simulink model "VSG_2M"  (R2022b)
settings: Solver=FixedStepAuto  StartTime=0.0  StopTime=2  FixedStep=1e-6  RelTol=1e-3
model workspace (MAT data in the model file):
  C = 0.0003
  D = 500
  GP = 0.6
  GQ = 20
  J = 2
  KQ = 0.06
  Kf = 80000
  Kv = 577
  L = 0.001
  Pref = 2000000
  Qref = 0
  Ts = 0.0001
  Ts_Power = 1e-06
  Ug = 400
  Vdc = 1000
  fsw = 20000
  t0 = 0.5
  tco = 1.3
  tf = 1.2
  wn = 314.159265359
undefined symbols (not defined in the file): DiscIntNeverNeededParam, Ion, Lithium
libraries: spsSeriesRLCBranchLib x8, spsFirstOrderFilterLib x7, spsMeanLib x5, slpidlib x5, spsabctodq0Lib x4, spsStairGeneratorLib x4, spsDiodeLib x4, spsPWMGeneratorDCDCLib x3, spsThreePhaseVIMeasurementLib x3, spsThreePhaseSeriesRLCBranchLib x3, spsPowerPositiveSequenceLib x2, spsBoostConverterLib x2
(part 1 of 2)
settings Model: SimulationMode=accelerator  Creator=刘明炜  LastModifiedBy=刘明炜
settings DataIOCC: ReturnWorkspaceOutputs=off

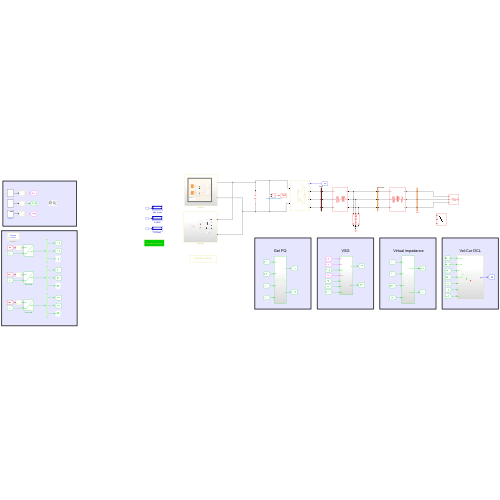
[thumbnail: Simulink's stored preview of the top-level diagram]
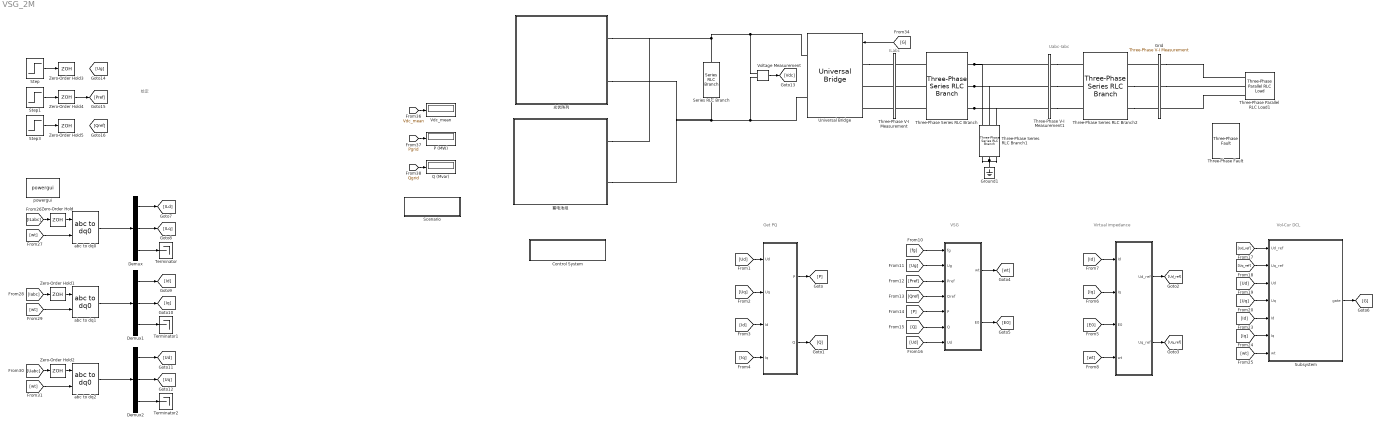
== system VSG_2M ==
  note: 给定
  note: ILabc
  note: VSG
  note: Get PQ
  note: Virtual impedance
  note: Vol-Cur DCL
  note: Uabc-Iabc
  " " : Subsystem
  "  " : Subsystem
  "   " : Subsystem
  Control System : Subsystem
      mask Display: disp('CONTROL SYSTEM')
  Demux : Demux  Outputs=3
  Demux1 : Demux  Outputs=3
  Demux2 : Demux  Outputs=3
  Grid : spsThreePhaseVIMeasurementLib/Three-Phase V-I Measurement  VoltageMeasurement=phase-to-ground  SetLabelV=on  LabelV=Vgrid  Vpu=off  VpuLL=off  CurrentMeasurement=yes  SetLabelI=on  LabelI=Igrid  Ipu=off  Pbase=100e6  Vbase=500e3  OutputType=Complex  PhasorSimulation=off  PSBequivalent=0
  Ground1 : spsGroundLib/Ground  LConnTagsString=a
  P (MW) : Display
      settings: Format=bank  Decimation=200
  Q (Mvar) : Display
      settings: Format=bank  Decimation=200
  Scenario : Subsystem
      mask Display: disp('Scenario & Scopes')
  Series RLC Branch : spsSeriesRLCBranchLib/Series RLC Branch  LConnTagsString=__new0  RConnTagsString=__new0  BranchType=C  Resistance=1  Inductance=1e-3  SetiL0=off  InitialCurrent=0  Capacitance=0.47  Setx0=off  InitialVoltage=0  Measurements=None
  Step : Step  Time=t0  Before=1  After=Ug  SampleTime=0
  Step1 : Step  Time=0  After=Pref  SampleTime=0
  Step3 : Step  Time=0  After=Qref  SampleTime=0
  Subsystem : Subsystem
  Terminator : Terminator
  Terminator1 : Terminator
  Terminator2 : Terminator
  Three-Phase Parallel RLC Load1 : spsThreePhaseParallelRLCLoadLib/Three-Phase Parallel RLC Load  LConnTagsString=A|B|C  Configuration=Y (grounded)  NominalVoltage=400  Vabc=[1e3 1e3 1e3]  Vabcp=[1e3 1e3 1e3]  NominalFrequency=50  UnbalancedPower=off  ActivePower=Pref  InductivePower=0  CapacitivePower=0  Pabc=[10e3 9e3 11e3]  QLabc=[100 90 110]  QCabc=[100 90 110]  Pabcp=[10e3 9e3 11e3]  QLabcp=[100 90 110]  QCabcp=[100 90 110]  Measurements=Branch voltages and currents  LoadType=constant Z
  Three-Phase Series RLC Branch : spsThreePhaseSeriesRLCBranchLib/Three-Phase Series RLC Branch  LConnTagsString=A|B|C  RConnTagsString=A|B|C  BranchType=RL  Resistance=0  Inductance=L  Capacitance=0  Measurements=None
  Three-Phase Series RLC Branch1 : spsThreePhaseSeriesRLCBranchLib/Three-Phase Series RLC Branch  LConnTagsString=A|B|C  RConnTagsString=A|B|C  BranchType=RLC  Resistance=1  Inductance=0  Capacitance=C  Measurements=None
  Three-Phase Series RLC Branch2 : spsThreePhaseSeriesRLCBranchLib/Three-Phase Series RLC Branch  LConnTagsString=A|B|C  RConnTagsString=A|B|C  BranchType=RLC  Resistance=0  Inductance=0.00000001  Capacitance=0  Measurements=None
  Three-Phase V-I Measurement : spsThreePhaseVIMeasurementLib/Three-Phase V-I Measurement  VoltageMeasurement=phase-to-phase  SetLabelV=on  LabelV=Vinv  Vpu=off  VpuLL=off  CurrentMeasurement=yes  SetLabelI=on  LabelI=ILabc  Ipu=off  Pbase=100e6  Vbase=500e3  OutputType=Complex  PhasorSimulation=off  PSBequivalent=0
  Three-Phase V-I Measurement1 : spsThreePhaseVIMeasurementLib/Three-Phase V-I Measurement  VoltageMeasurement=phase-to-ground  SetLabelV=on  LabelV=Uabc  Vpu=off  VpuLL=off  CurrentMeasurement=yes  SetLabelI=on  LabelI=Iabc  Ipu=off  Pbase=100e6  Vbase=500e3  OutputType=Complex  PhasorSimulation=off  PSBequivalent=0
  Three-Phase Fault : spsThreePhaseFaultLib/Three-Phase Fault  InitialStates=0  FaultA=on  FaultB=off  FaultC=off  GroundFault=on  SwitchTimes=[tf tco]  External=off  SwitchStatus=NaN  FaultResistance=1  GroundResistance=0.01  SnubberResistance=1e6  SnubberCapacitance=inf  Measurements=Fault voltages and currents
  Universal Bridge : spsUniversalBridgeLib/Universal Bridge  Arms=3  SnubberResistance=1e5  SnubberCapacitance=inf  Device=IGBT / Diodes  Ron=0.001  Lon=0  ForwardVoltages="[  0  0  ]"  ForwardVoltage=0  GTOparameters=[ 10e-6 , 20e-6 ]  IGBTparameters=[ 1e-6 , 2e-6 ]  Measurements=None  Measurements_2=None  converterType=Rectifier
  Vdc_mean : Display
      settings: Decimation=200
  Voltage Measurement : spsVoltageMeasurementLib/Voltage Measurement  PhasorSimulation=off  OutputType=Complex  PSBequivalent=0
  Zero-Order Hold{,1..5} (6 alike) : ZeroOrderHold  SampleTime=1/fsw
  abc to dq0 : spsabctodq0Lib/abc to dq0  Alignment=90 degrees behind phase A axis
  abc to dq1 : spsabctodq0Lib/abc to dq0  Alignment=90 degrees behind phase A axis
  abc to dq2 : spsabctodq0Lib/abc to dq0  Alignment=90 degrees behind phase A axis
  powergui : spspowerguiLib/powergui  Priority=1  SimulationMode=Discrete  SampleTime=Ts_Power  frequency=60  Iterations=50  frequencyindice=0  Pbase=100e6  ErrMax=1e-4  UnitsV=kV  UnitsW=MW  buscounter=0  FunctionMessages=off  echomessages=off  EnableUseOfTLC=off  CurrentSourceSwitches=off  DisableSnubberDevices=off  DisableRonSwitches=off  DisableVfSwitches=off  DisplayEquations=off  AutomaticDiscreteSolvers=off  SolverType=Tustin/Backward Euler (TBE)  Interpol=off  ExternalGateDelay=off  methode=off  Ts=100  x0status=blocks  SPID=on  SwTol=0  HookPort=off  NonlinearTolerance=1e-4  nMaxIteration=100  ContinueOnMaxIteration=off  RestoreLinks=warning  ResistiveCurrentMeasurement=off  Frange=[0:2:500]  Ylog=off  Xlog=on  ShowGrid=off  save=off  variable=ZData  structure=0  ZoomFFT=off  StartTime=0.0  cycles=1  DisplayStyle=1  fundamental=60  FreqAxis=off  MaxFrequency=1000  frequencyindicesteady=1  RmsSteady=1  display=off
  光伏阵列 : Subsystem
  蓄电池组 : Subsystem
  wires:
  [Id] -> " "/3(Id)
  [Iq] -> " "/4(Iq)
  [Uq] -> " "/2(Uq)
  " "/1(P) -> [P]
  [Ud] -> " "/1(Ud)
  " "/2(Q) -> [Q]
  [E0] -> "   "/3(E0)
  [Iq] -> "   "/2(Iq)
  [Id] -> "   "/1(Id)
  [wt] -> "   "/4(wt)
  "   "/1(Ud_ref) -> [Ud_ref]
  "   "/2(Uq_ref) -> [Uq_ref]
  [Qref] -> "  "/4(Qref)
  [Ud] -> "  "/7(Ud)
  [fg] -> "  "/1(fg)
  "  "/2(E0) -> [E0]
  [Q] -> "  "/6(Q)
  [P] -> "  "/5(P)
  [Ug] -> "  "/2(Ug)
  [Pref] -> "  "/3(Pref)
  "  "/1(wt) -> [wt]
  [Ud] -> Subsystem/3(Ud)
  Subsystem/1(gate) -> [G]
  [wt] -> Subsystem/7(wt)
  [Ud_ref] -> Subsystem/1(Ud_ref)
  [Uq_ref] -> Subsystem/2(Uq_ref)
  [Iq] -> Subsystem/6(Iq)
  [Uq] -> Subsystem/4(Uq)
  [Id] -> Subsystem/5(Id)
  abc to dq0/1 -> Demux/1
  Demux/1 -> [ILd]
  Demux/2 -> [ILq]
  Demux/3 -> Terminator/1
  Demux1/2 -> [Iq]
  Demux1/1 -> [Id]
  abc to dq1/1 -> Demux1/1
  Demux1/3 -> Terminator1/1
  Demux2/2 -> [Uq]
  Demux2/1 -> [Ud]
  abc to dq2/1 -> Demux2/1
  Demux2/3 -> Terminator2/1
  Zero-Order Hold/1 -> abc to dq0/1
  [ILabc] -> Zero-Order Hold/1
  [Iabc] -> Zero-Order Hold1/1
  Zero-Order Hold1/1 -> abc to dq1/1
  [Uabc] -> Zero-Order Hold2/1
  Zero-Order Hold2/1 -> abc to dq2/1
  [wt] -> abc to dq0/2
  [wt] -> abc to dq1/2
  [wt] -> abc to dq2/2
  Step/1 -> Zero-Order Hold3/1
  Step1/1 -> Zero-Order Hold4/1
  [G] -> Universal Bridge/1
  Step3/1 -> Zero-Order Hold5/1
  [Qgrid] -> Q (Mvar)/1
  [Pgrid] -> P (MW)/1
  [Vdc_mean] -> Vdc_mean/1
  Voltage Measurement/1 -> [Vdc]
  Zero-Order Hold4/1 -> [Pref]
  connections:
  Three-Phase Series RLC Branch/RConn1 -- Three-Phase Series RLC Branch1/LConn1 -- Three-Phase V-I Measurement1/LConn1
  Ground1/LConn1 -- Three-Phase Series RLC Branch1/RConn2 -- Three-Phase Series RLC Branch1/RConn3 -- Three-Phase Series RLC Branch1/RConn1
  Three-Phase Series RLC Branch/RConn3 -- Three-Phase V-I Measurement1/LConn3 -- Three-Phase Series RLC Branch1/LConn3
  Three-Phase Series RLC Branch/RConn2 -- Three-Phase Series RLC Branch1/LConn2 -- Three-Phase V-I Measurement1/LConn2
  Three-Phase Series RLC Branch/LConn1 -- Three-Phase V-I Measurement/RConn1
  Three-Phase V-I Measurement1/RConn3 -- Three-Phase Series RLC Branch2/LConn3
  Three-Phase V-I Measurement/LConn2 -- Universal Bridge/LConn2
  Universal Bridge/RConn2 -- Voltage Measurement/LConn2 -- 蓄电池组/RConn2 -- 光伏阵列/RConn2 -- Series RLC Branch/RConn1
  Universal Bridge/LConn1 -- Three-Phase V-I Measurement/LConn1
  Three-Phase V-I Measurement1/RConn2 -- Three-Phase Series RLC Branch2/LConn2
  Universal Bridge/RConn1 -- 蓄电池组/RConn1 -- 光伏阵列/RConn1 -- Series RLC Branch/LConn1 -- Voltage Measurement/LConn1
  Three-Phase V-I Measurement1/RConn1 -- Three-Phase Series RLC Branch2/LConn1
  Three-Phase Series RLC Branch/LConn2 -- Three-Phase V-I Measurement/RConn2
  Three-Phase Series RLC Branch/LConn3 -- Three-Phase V-I Measurement/RConn3
  Three-Phase V-I Measurement/LConn3 -- Universal Bridge/LConn3
  Grid/LConn1 -- Three-Phase Series RLC Branch2/RConn1
  Three-Phase Series RLC Branch2/RConn2 -- Grid/LConn2
  Three-Phase Series RLC Branch2/RConn3 -- Grid/LConn3
  Grid/RConn1 -- Three-Phase Parallel RLC Load1/LConn1
  Grid/RConn2 -- Three-Phase Parallel RLC Load1/LConn2
  Three-Phase Parallel RLC Load1/LConn3 -- Grid/RConn3

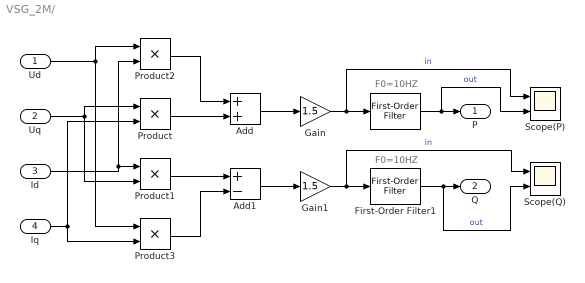
== system VSG_2M/  ==
  note: F0=10HZ
  note: F0=10HZ
  Ud : Inport
  Uq : Inport  Port=2
  Id : Inport  Port=3
  Iq : Inport  Port=4
  " " : spsFirstOrderFilterLib/First-Order Filter  FilterType=Lowpass  Tc=10e-3  Ts=1/fsw  Initialize=on  Vac_Init=[0, 0, 10]  Vdc_Init=0  PlotResponse=off  FreqRange="[0,  200,  1]"
  Add : Sum
  Add1 : Sum  Inputs=+-
  First-Order Filter1 : spsFirstOrderFilterLib/First-Order Filter  FilterType=Lowpass  Tc=10e-3  Ts=1/fsw  Initialize=on  Vac_Init=[0, 0, 10]  Vdc_Init=0  PlotResponse=off  FreqRange="[0,  200,  1]"
  Gain : Gain  Gain=1.5
  Gain1 : Gain  Gain=1.5
  Product{,1..3} (4 alike) : Product
  Scope(P) : Scope  NumInputPorts=2
  Scope(Q) : Scope  NumInputPorts=2
  P : Outport
  Q : Outport  Port=2
  wires:
  Gain1/1 -> First-Order Filter1/1, Scope(Q)/1  "in"
  Product2/1 -> Add/1
  " "/1 -> Scope(P)/2, P/1  "out"
  Add1/1 -> Gain1/1
  Gain/1 -> " "/1, Scope(P)/1  "in"
  First-Order Filter1/1 -> Scope(Q)/2, Q/1  "out"
  Product/1 -> Add/2
  Product3/1 -> Add1/2
  Product1/1 -> Add1/1
  Ud/1 -> Product3/1, Product2/1
  Add/1 -> Gain/1
  Id/1 -> Product1/1, Product2/2
  Iq/1 -> Product3/2, Product/2
  Uq/1 -> Product1/2, Product/1

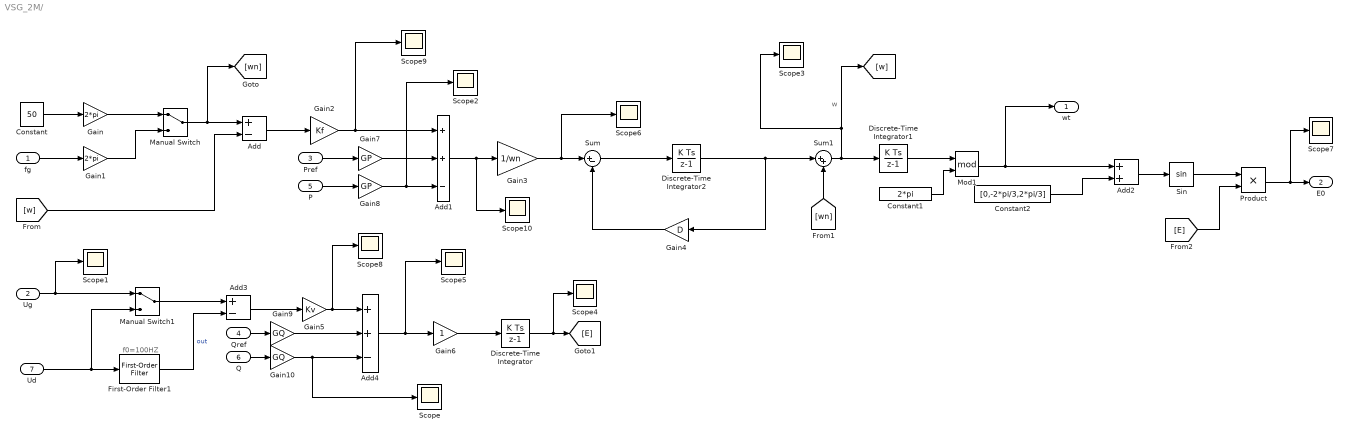
== system VSG_2M/   ==
  note: f0=100HZ
  note: w
  fg : Inport
  Ug : Inport  Port=2
  Pref : Inport  Port=3
  Qref : Inport  Port=4
  P : Inport  Port=5
  Q : Inport  Port=6
  Ud : Inport  Port=7
  Add : Sum  Inputs=+-
  Add1 : Sum  Inputs=++-
  Add2 : Sum
  Add3 : Sum  Inputs=+-
  Add4 : Sum  Inputs=++-
  Constant : Constant  Value=50
  Constant1 : Constant  Value=2*pi
  Constant2 : Constant  Value=[0,-2*pi/3,2*pi/3]
  Discrete-Time Integrator : DiscreteIntegrator  gainval=KQ  SampleTime=1/fsw  ICPrevOutput=DiscIntNeverNeededParam  ICPrevScaledInput=DiscIntNeverNeededParam
  Discrete-Time Integrator1 : DiscreteIntegrator  SampleTime=1/fsw  ICPrevOutput=DiscIntNeverNeededParam  ICPrevScaledInput=DiscIntNeverNeededParam
  Discrete-Time Integrator2 : DiscreteIntegrator  gainval=1/J  SampleTime=1/fsw  ICPrevOutput=DiscIntNeverNeededParam  ICPrevScaledInput=DiscIntNeverNeededParam
  First-Order Filter1 : spsFirstOrderFilterLib/First-Order Filter  FilterType=Lowpass  Tc=10e-3  Ts=1/fsw  Initialize=on  Vac_Init=[0, 0, 10]  Vdc_Init=0  PlotResponse=off  FreqRange="[0,  200,  1]"
  Gain : Gain  Gain=2*pi
  Gain1 : Gain  Gain=2*pi
  Gain10 : Gain  Gain=GQ
  Gain2 : Gain  Gain=Kf
  Gain3 : Gain  Gain=1/wn
  Gain4 : Gain  Gain=D
  Gain5 : Gain  Gain=Kv
  Gain6 : Gain
  Gain7 : Gain  Gain=GP
  Gain8 : Gain  Gain=GP
  Gain9 : Gain  Gain=GQ
  Manual Switch : ManualSwitch
  Manual Switch1 : ManualSwitch
  Mod1 : Math  Operator=mod
  Product : Product
  Scope{,1..10} (11 alike) : Scope
  Sin : Trigonometry
  Sum : Sum  Inputs=|+-
  Sum1 : Sum  Inputs=|++
  wt : Outport
  E0 : Outport  Port=2
  wires:
  Ug/1 -> Scope1/1, Manual Switch1/1
  Gain3/1 -> Scope6/1, Sum/1
  Gain2/1 -> Scope9/1, Add1/1
  Product/1 -> Scope7/1, E0/1
  Add/1 -> Gain2/1
  Manual Switch1/1 -> Add3/1
  [E] -> Product/2
  Add4/1 -> Scope5/1, Gain6/1
  Mod1/1 -> wt/1, Add2/1
  Sum1/1 -> Discrete-Time Integrator1/1, Scope3/1, [w]
  fg/1 -> Gain1/1
  Constant2/1 -> Add2/2
  First-Order Filter1/1 -> Add3/2  "out"
  Ud/1 -> First-Order Filter1/1, Manual Switch1/2
  Constant/1 -> Gain/1
  Sin/1 -> Product/1
  Add2/1 -> Sin/1
  Gain4/1 -> Sum/2
  P/1 -> Gain8/1
  Gain/1 -> Manual Switch/1
  Gain1/1 -> Manual Switch/2
  Discrete-Time Integrator2/1 -> Gain4/1, Sum1/1
  Constant1/1 -> Mod1/2
  Gain5/1 -> Scope8/1, Add4/1
  Q/1 -> Gain10/1
  Manual Switch/1 -> [wn], Add/1
  Pref/1 -> Gain7/1
  Add1/1 -> Scope10/1, Gain3/1
  Add3/1 -> Gain5/1
  Gain6/1 -> Discrete-Time Integrator/1
  Qref/1 -> Gain9/1
  [wn] -> Sum1/2
  Sum/1 -> Discrete-Time Integrator2/1
  Discrete-Time Integrator/1 -> Scope4/1, [E]
  Discrete-Time Integrator1/1 -> Mod1/1
  [w] -> Add/2
  Gain7/1 -> Add1/2
  Gain8/1 -> Scope2/1, Add1/3
  Gain9/1 -> Add4/2
  Gain10/1 -> Scope/1, Add4/3

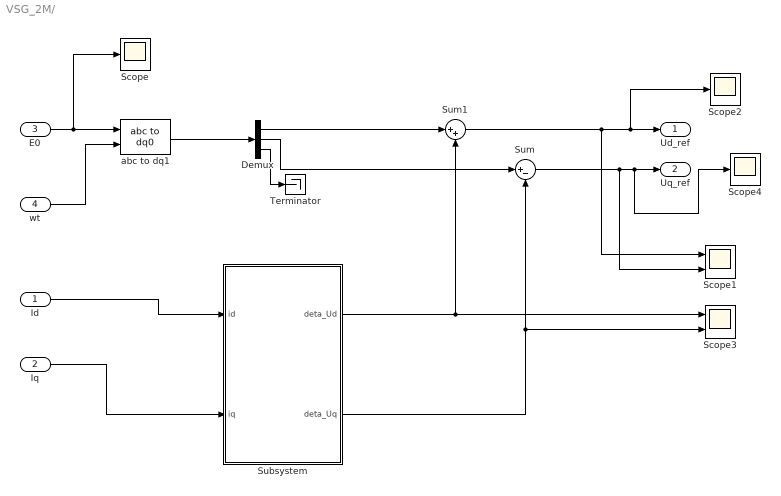
== system VSG_2M/    ==
  Id : Inport
  Iq : Inport  Port=2
  E0 : Inport  Description=Cont  Port=3
  wt : Inport  Port=4
  Demux : Demux  Outputs=3
  Scope : Scope
  Scope1 : Scope  NumInputPorts=2
  Scope2 : Scope
  Scope3 : Scope  NumInputPorts=2
  Scope4 : Scope
  Subsystem : Subsystem
  Sum : Sum  Inputs=|+-
  Sum1 : Sum  Inputs=|++
  Terminator : Terminator
  abc to dq1 : spsabctodq0Lib/abc to dq0  Alignment=90 degrees behind phase A axis
  Ud_ref : Outport
  Uq_ref : Outport  Port=2
  wires:
  Demux/1 -> Sum1/1
  E0/1 -> Scope/1, abc to dq1/1
  Id/1 -> Subsystem/1(id)
  abc to dq1/1 -> Demux/1
  Subsystem/2(deta_Uq) -> Sum/2, Scope3/2
  Sum1/1 -> Scope2/1, Ud_ref/1, Scope1/1
  wt/1 -> abc to dq1/2
  Demux/2 -> Sum/1
  Subsystem/1(deta_Ud) -> Sum1/2, Scope3/1
  Iq/1 -> Subsystem/2(iq)
  Sum/1 -> Scope4/1, Uq_ref/1, Scope1/2
  Demux/3 -> Terminator/1

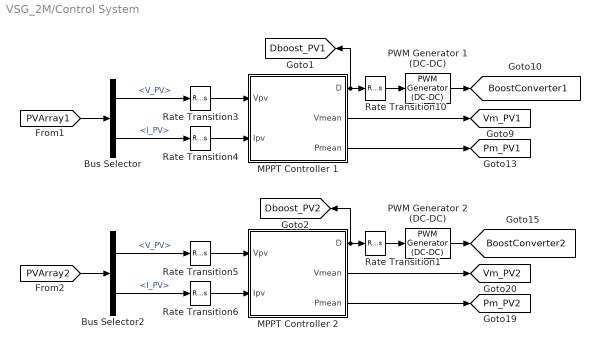
== system VSG_2M/Control System ==
  Bus Selector : BusSelector  OutputSignals=V_PV,I_PV
  Bus Selector2 : BusSelector  OutputSignals=V_PV,I_PV
  MPPT Controller 1 : Subsystem  mask(MPPT Controller - Perturb and Observe algorithm (PandO)){Dinit=0.35, Dlimits=[0.8, 0.3], deltaD=60e-6, Fc=1000, Ts=Ts}
      mask prompts: Dinit "Duty cycle (D) initial value"; Dlimits "D limits [Upper, Lower]"; deltaD "Increment value for PandO algorithm"; Fc "Measurement filter cutoff frequency (Hz)"; Ts "Sample time (s)"
      mask init:
      | Dmax=Dlimits(1);
      | Dmin=Dlimits(2);
  MPPT Controller 2 : Subsystem  mask(MPPT Controller - Perturb and Observe algorithm (PandO)){Dinit=0.55, Dlimits=[0.8, 0.47], deltaD=60e-6, Fc=1000, Ts=Ts}
      mask prompts: Dinit "Duty cycle (D) initial value"; Dlimits "D limits [Upper, Lower]"; deltaD "Increment value for PandO algorithm"; Fc "Measurement filter cutoff frequency (Hz)"; Ts "Sample time (s)"
      mask init:
      | Dmax=Dlimits(1);
      | Dmin=Dlimits(2);
  PWM Generator 1 (DC-DC) : spsPWMGeneratorDCDCLib/PWM Generator (DC-DC)  Fsw=5000  Ts=Ts_Power
  PWM Generator 2 (DC-DC) : spsPWMGeneratorDCDCLib/PWM Generator (DC-DC)  Fsw=5000  Ts=Ts_Power
  Rate Transition1 : RateTransition  OutPortSampleTime=Ts_Power
  Rate Transition10 : RateTransition  OutPortSampleTime=Ts_Power
  Rate Transition{3..6} (4 alike) : RateTransition  OutPortSampleTime=Ts
  tag scope: BoostConverter1=global, BoostConverter2=global, Dboost_PV1=global, Dboost_PV2=global, Pm_PV1=global, Pm_PV2=global, Vm_PV1=global, Vm_PV2=global
  wires:
  MPPT Controller 2/2(Vmean) -> [Vm_PV2]
  Bus Selector2/1 -> Rate Transition5/1  "<V_PV>"
  Rate Transition3/1 -> MPPT Controller 1/1(Vpv)
  Rate Transition4/1 -> MPPT Controller 1/2(Ipv)
  Bus Selector/2 -> Rate Transition4/1  "<I_PV>"
  MPPT Controller 2/3(Pmean) -> [Pm_PV2]
  MPPT Controller 1/1(D) -> [Dboost_PV1], Rate Transition10/1
  Bus Selector/1 -> Rate Transition3/1  "<V_PV>"
  Bus Selector2/2 -> Rate Transition6/1  "<I_PV>"
  Rate Transition1/1 -> PWM Generator 2 (DC-DC)/1
  Rate Transition6/1 -> MPPT Controller 2/2(Ipv)
  MPPT Controller 1/3(Pmean) -> [Pm_PV1]
  MPPT Controller 1/2(Vmean) -> [Vm_PV1]
  Rate Transition10/1 -> PWM Generator 1 (DC-DC)/1
  MPPT Controller 2/1(D) -> [Dboost_PV2], Rate Transition1/1
  Rate Transition5/1 -> MPPT Controller 2/1(Vpv)
  PWM Generator 1 (DC-DC)/1 -> [BoostConverter1]
  PWM Generator 2 (DC-DC)/1 -> [BoostConverter2]
  [PVArray1] -> Bus Selector/1
  [PVArray2] -> Bus Selector2/1

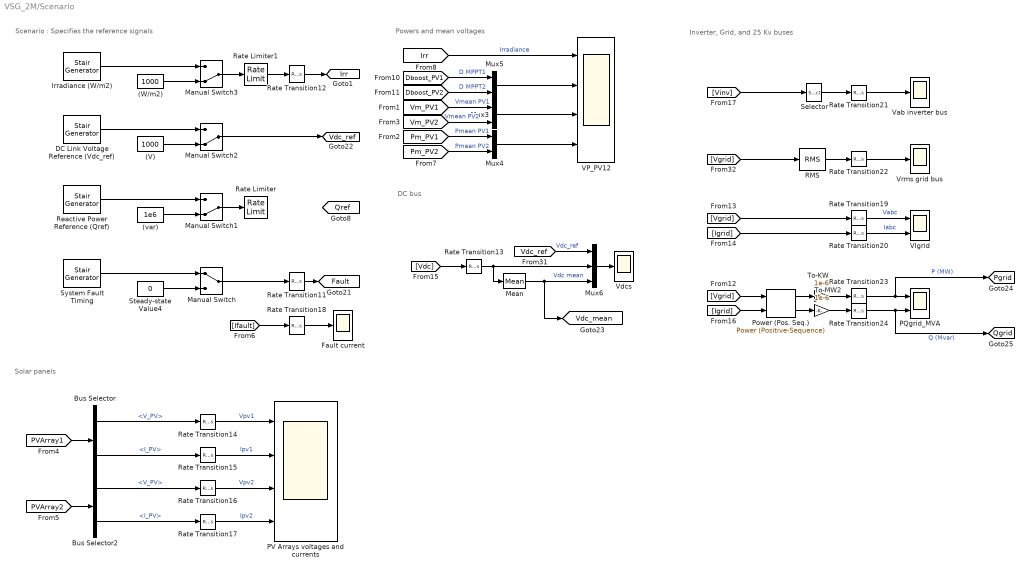
== system VSG_2M/Scenario ==
  note: DC bus
  note: Powers and mean voltages
  note: Inverter, Grid, and 25 Kv buses
  note: Solar panels
  note: Scenario : Specifies the reference signals
  (V) : Constant  Value=1000
  (W/m2) : Constant  Value=1000
  (var) : Constant  Value=1e6
  Bus Selector : BusSelector  OutputSignals=V_PV,I_PV
  Bus Selector2 : BusSelector  OutputSignals=V_PV,I_PV
  DC Link Voltage Reference (Vdc_ref) : spsStairGeneratorLib/Stair Generator  t=[0, 0.2, 0.4]  e=[1000, 1050, 1000]  Ts=Ts
  Fault current : Scope
  Irradiance (W/m2) : spsStairGeneratorLib/Stair Generator  t=[0, 0.2, 0.4]  e=[1000, 250,1000]  Ts=Ts
  Manual Switch : ManualSwitch
  Manual Switch1 : ManualSwitch  CurrentSetting=0
  Manual Switch2 : ManualSwitch  CurrentSetting=0
  Manual Switch3 : ManualSwitch  CurrentSetting=0
  Mean : spsMeanLib/Mean  Freq=60  Vinit=1000  Ts=Ts
  Mux3 : Mux  Inputs=2
  Mux4 : Mux  Inputs=2
  Mux5 : Mux  Inputs=2
  Mux6 : Mux  Inputs=3
  PQgrid_MVA : Scope  NumInputPorts=2
  PV Arrays voltages and currents : Scope  NumInputPorts=4
  Power (Pos. Seq.) : spsPowerPositiveSequenceLib/Power (Positive-Sequence)  Freq=50  Vinit=[20570,-37]  Iinit=[70, -63]  Ts=Ts_Power
      settings: LibrarySourceBlock=|
      | sps_lib/Sensors and Measurements/Power
      | (Positive-Sequence)
  RMS : spsRMSLib/RMS  TrueRMS=off  Freq=50  RMSInit=25000  Ts=Ts_Power
  Rate Limiter : RateLimiter  RisingSlewLimit=1e6/(1/60)  FallingSlewLimit=-1e6/(1/60)  SampleTimeMode=inherited  InitialCondition=1e6
  Rate Limiter1 : RateLimiter  RisingSlewLimit=1000/(1/60)  FallingSlewLimit=-1000/(1/60)  SampleTimeMode=inherited  InitialCondition=1000
  Rate Transition11 : RateTransition  OutPortSampleTime=Ts_Power
  Rate Transition12 : RateTransition  OutPortSampleTime=Ts_Power
  Rate Transition{13..24} (12 alike) : RateTransition  OutPortSampleTime=Ts
  "Reactive Power Reference (Qref) " : spsStairGeneratorLib/Stair Generator  t=[0, 0.2, 0.4]  e=[1e6, -1e6, 1e6]  Ts=Ts
  Selector : Selector  InputPortWidth=3  IndexOptions=Index vector (dialog)  Indices=1  OutputSizes=1
  Steady-state Value4 : Constant  Value=0
  System Fault Timing : spsStairGeneratorLib/Stair Generator  t=[0, 0.25, 0.45]  e=[0, 1, 0]  Ts=Ts
  To-KW : Gain  Gain=1e-6
  To-MW2 : Gain  Gain=1e-6
  VIgrid : Scope  NumInputPorts=2
  VP_PV12 : Scope  NumInputPorts=4
  Vab inverter bus : Scope
  Vdcs : Scope
  Vrms grid bus : Scope
  tag scope: Fault=global, Irr=global, Pgrid=global, Qgrid=global, Qref=global, Vdc_mean=global, Vdc_ref=global
  wires:
  (W/m2)/1 -> Manual Switch3/2
  (V)/1 -> Manual Switch2/2
  Steady-state Value4/1 -> Manual Switch/2
  DC Link Voltage Reference (Vdc_ref)/1 -> Manual Switch2/1
  System Fault Timing/1 -> Manual Switch/1
  Manual Switch/1 -> Rate Transition11/1
  Rate Limiter1/1 -> Rate Transition12/1
  (var)/1 -> Manual Switch1/2
  "Reactive Power Reference (Qref) "/1 -> Manual Switch1/1
  Manual Switch1/1 -> Rate Limiter/1
  Manual Switch2/1 -> [Vdc_ref]
  Irradiance (W/m2)/1 -> Manual Switch3/1
  Manual Switch3/1 -> Rate Limiter1/1
  Rate Transition12/1 -> [Irr]
  Bus Selector2/1 -> Rate Transition16/1  "<V_PV>"
  Bus Selector/2 -> Rate Transition15/1  "<I_PV>"
  Bus Selector/1 -> Rate Transition14/1  "<V_PV>"
  Rate Transition19/1 -> VIgrid/1  "Vabc"
  [Pm_PV1] -> Mux4/1  "Pmean PV1"
  Rate Transition17/1 -> PV Arrays voltages and currents/4  "Ipv2"
  RMS/1 -> Rate Transition22/1
  [Pm_PV2] -> Mux4/2  "Pmean PV2"
  [Irr] -> VP_PV12/1  "Irradiance"
  Rate Transition22/1 -> Vrms grid bus/1
  Rate Transition16/1 -> PV Arrays voltages and currents/3  "Vpv2"
  Mux3/1 -> VP_PV12/3
  [Vgrid] -> RMS/1
  [Vgrid] -> Power (Pos. Seq.)/1
  Rate Transition23/1 -> [Pgrid], PQgrid_MVA/1  "P (MW)"
  [PVArray1] -> Bus Selector/1
  Rate Transition20/1 -> VIgrid/2  "Iabc"
  Mux6/1 -> Vdcs/1
  Mux4/1 -> VP_PV12/4
  Rate Transition15/1 -> PV Arrays voltages and currents/2  "Ipv1"
  Mux5/1 -> VP_PV12/2
  Power (Pos. Seq.)/2 -> To-MW2/1
  [Igrid] -> Rate Transition20/1
  Rate Transition18/1 -> Fault current/1
  [Vm_PV2] -> Mux3/2  "Vmean PV2"
  Rate Transition14/1 -> PV Arrays voltages and currents/1  "Vpv1"
  [Vgrid] -> Rate Transition19/1
  Rate Transition13/1 -> Mean/1, Mux6/2
  Power (Pos. Seq.)/1 -> To-KW/1
  [Dboost_PV1] -> Mux5/1  "D MPPT1"
  [Vinv] -> Selector/1
  Mean/1 -> Mux6/3, [Vdc_mean]  "Vdc mean"
  Rate Transition11/1 -> [Fault]
  [Dboost_PV2] -> Mux5/2  "D MPPT2"
  [Vm_PV1] -> Mux3/1  "Vmean PV1"
  [Vdc_ref] -> Mux6/1  "Vdc_ref"
  [Igrid] -> Power (Pos. Seq.)/2
  Bus Selector2/2 -> Rate Transition17/1  "<I_PV>"
  Rate Transition24/1 -> [Qgrid], PQgrid_MVA/2  "Q (Mvar)"
  [Vdc] -> Rate Transition13/1
  [PVArray2] -> Bus Selector2/1
  [Ifault] -> Rate Transition18/1
  Selector/1 -> Rate Transition21/1
  Rate Transition21/1 -> Vab inverter bus/1
  To-MW2/1 -> Rate Transition24/1
  To-KW/1 -> Rate Transition23/1

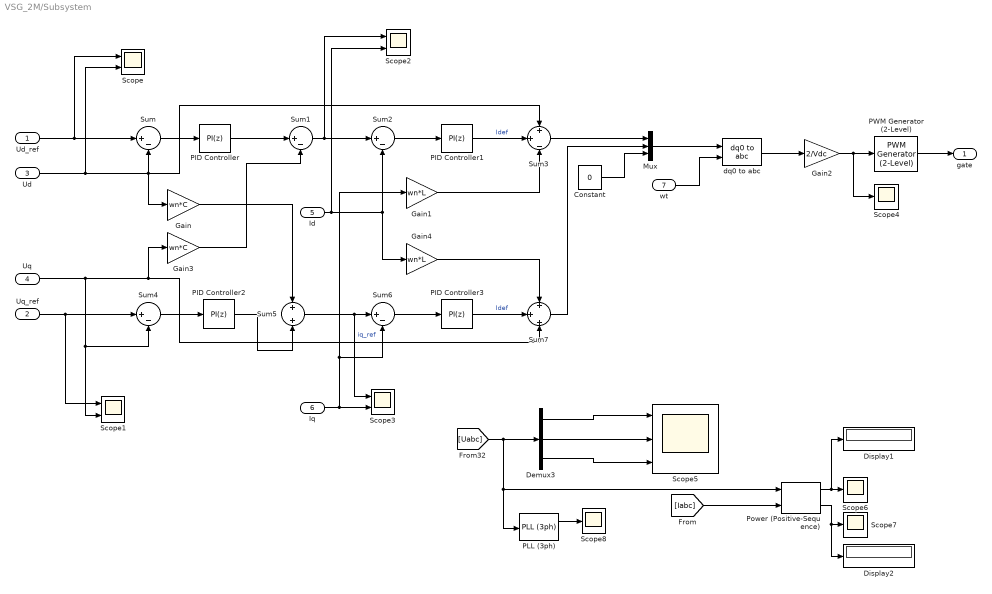
== system VSG_2M/Subsystem ==
  Ud_ref : Inport
  Uq_ref : Inport  Port=2
  Ud : Inport  Port=3
  Uq : Inport  Port=4
  Id : Inport  Port=5
  Iq : Inport  Port=6
  wt : Inport  Port=7
  Constant : Constant  Value=0
  Demux3 : Demux  Outputs=3
  Display1 : Display
  Display2 : Display
  Gain : Gain  Gain=wn*C
  Gain1 : Gain  Gain=wn*L
  Gain2 : Gain  Gain=2/Vdc
  Gain3 : Gain  Gain=wn*C
  Gain4 : Gain  Gain=wn*L
  Mux : Mux  Inputs=3
  PID Controller : slpidlib/PID Controller  Controller=PI  Form=Parallel  TimeDomain=Discrete-time  UseExternalTs=off  SampleTime=-1  IntegratorMethod=Forward Euler  FilterMethod=Forward Euler  ControllerParametersSource=internal  P=10  I=50  UseKiTs=off  D=0  N=100  UseFilter=on  TunerSelectOption=Transfer Function Based (PID Tuner App)  InitialConditionSource=internal  InitialConditionForIntegrator=0  InitialConditionForFilter=0  DifferentiatorICPrevScaledInput=0  ExternalReset=none  TrackingMode=off  Kt=1  LimitOutput=off  SatLimitsSource=internal  UpperSaturationLimit=inf  LowerSaturationLimit=-inf  LinearizeAsGain=on  AntiWindupMode=none  Kb=1  LimitIntegrator=off  UpperIntegratorSaturationLimit=inf  LowerIntegratorSaturationLimit=-inf  POutMin=[]  POutMax=[]  IOutMin=[]  IOutMax=[]  DOutMin=[]  DOutMax=[]  NOutMin=[]  NOutMax=[]  SumOutMin=[]  SumOutMax=[]  SaturationOutMin=[]  SaturationOutMax=[]  PParamMin=[]  PParamMax=[]  IParamMin=[]  IParamMax=[]  DParamMin=[]  DParamMax=[]  NParamMin=[]  NParamMax=[]  KbParamMin=[]  KbParamMax=[]  KtParamMin=[]  KtParamMax=[]  KbOutMin=[]  KbOutMax=[]  KtOutMin=[]  KtOutMax=[]  IntegratorOutMin=[]  IntegratorOutMax=[]  FilterOutMin=[]  FilterOutMax=[]  SumI1OutMin=[]  SumI1OutMax=[]  SumI2OutMin=[]  SumI2OutMax=[]  SumI3OutMin=[]  SumI3OutMax=[]  SumI4OutMin=[]  SumI4OutMax=[]  SumDOutMin=[]  SumDOutMax=[]  DifferentiatorOutMin=[]  DifferentiatorOutMax=[]  FilterDiffOutCoefMin=[]  FilterDiffOutCoefMax=[]  ReciprocalOutMin=[]  ReciprocalOutMax=[]  SumDenOutMin=[]  SumDenOutMax=[]  SumNumOutMin=[]  SumNumOutMax=[]  DivideOutMin=[]  DivideOutMax=[]  UdiffTsProdOutMin=[]  UdiffTsProdOutMax=[]  NTsProdOutMin=[]  NTsProdOutMax=[]  UintegralTsProdOutMin=[]  UintegralTsProdOutMax=[]  UngainTsProdOutMin=[]  UngainTsProdOutMax=[]  ClampingZeroOutDataTypeStr=Inherit: Inherit via back propagation  ClampingZeroOutMin=[]  ClampingZeroOutMax=[]  FilterDenConstantOutDataTypeStr=Inherit: Inherit via back propagation  FilterDenConstantOutMin=[]  FilterDenConstantOutMax=[]  PCopyOutDataTypeStr=Inherit: Inherit via back propagation  PCopyOutMin=[]  PCopyOutMax=[]  NCopyOutDataTypeStr=Inherit: Inherit via back propagation  NCopyOutMin=[]  NCopyOutMax=[]  IntegratorContinuousStateAttributes=''  IntegratorStateMustResolveToSignalObject=off  IntegratorRTWStateStorageClass=Auto  FilterContinuousStateAttributes=''  FilterStateMustResolveToSignalObject=off  FilterRTWStateStorageClass=Auto  ParallelPVariant=InternalParameters  IdealPVariant=Disabled  IVariant=InternalParameters  DVariant=Disabled  IntegratorVariant=Discrete  SatVariant=Disabled  AWVariant=Passthrough  PCopyVariant=Disabled  TRVariant=Disabled  FdbkBlocksVariant=Forward  IdealPFdbkVariant=Disabled  SatFdbkVariant=Disabled  DerivativeFilterVariant=Disabled  NVariant=Disabled  NCopyVariant=Disabled_SignalSpec  FilterICVariant=Disabled  IntegratorICVariant=InternalICs  ExternalResetVariant=Disabled  TRSumVariant=Passthrough  SumFdbkVariant=Disabled  SumVariant=Sum_PI  TsampFilterVariant=InternalTs  TsampNgainVariant=Passthrough  TsampIntegralVariant=Passthrough  ExternalSaturationOutDataTypeStr=Inherit: Same as second input
  PID Controller1 : slpidlib/PID Controller  Controller=PI  Form=Parallel  TimeDomain=Discrete-time  UseExternalTs=off  SampleTime=-1  IntegratorMethod=Forward Euler  FilterMethod=Forward Euler  ControllerParametersSource=internal  P=20  I=50  UseKiTs=off  D=0  N=100  UseFilter=on  TunerSelectOption=Transfer Function Based (PID Tuner App)  InitialConditionSource=internal  InitialConditionForIntegrator=0  InitialConditionForFilter=0  DifferentiatorICPrevScaledInput=0  ExternalReset=none  TrackingMode=off  Kt=1  LimitOutput=off  SatLimitsSource=internal  UpperSaturationLimit=inf  LowerSaturationLimit=-inf  LinearizeAsGain=on  AntiWindupMode=none  Kb=1  LimitIntegrator=off  UpperIntegratorSaturationLimit=inf  LowerIntegratorSaturationLimit=-inf  POutMin=[]  POutMax=[]  IOutMin=[]  IOutMax=[]  DOutMin=[]  DOutMax=[]  NOutMin=[]  NOutMax=[]  SumOutMin=[]  SumOutMax=[]  SaturationOutMin=[]  SaturationOutMax=[]  PParamMin=[]  PParamMax=[]  IParamMin=[]  IParamMax=[]  DParamMin=[]  DParamMax=[]  NParamMin=[]  NParamMax=[]  KbParamMin=[]  KbParamMax=[]  KtParamMin=[]  KtParamMax=[]  KbOutMin=[]  KbOutMax=[]  KtOutMin=[]  KtOutMax=[]  IntegratorOutMin=[]  IntegratorOutMax=[]  FilterOutMin=[]  FilterOutMax=[]  SumI1OutMin=[]  SumI1OutMax=[]  SumI2OutMin=[]  SumI2OutMax=[]  SumI3OutMin=[]  SumI3OutMax=[]  SumI4OutMin=[]  SumI4OutMax=[]  SumDOutMin=[]  SumDOutMax=[]  DifferentiatorOutMin=[]  DifferentiatorOutMax=[]  FilterDiffOutCoefMin=[]  FilterDiffOutCoefMax=[]  ReciprocalOutMin=[]  ReciprocalOutMax=[]  SumDenOutMin=[]  SumDenOutMax=[]  SumNumOutMin=[]  SumNumOutMax=[]  DivideOutMin=[]  DivideOutMax=[]  UdiffTsProdOutMin=[]  UdiffTsProdOutMax=[]  NTsProdOutMin=[]  NTsProdOutMax=[]  UintegralTsProdOutMin=[]  UintegralTsProdOutMax=[]  UngainTsProdOutMin=[]  UngainTsProdOutMax=[]  ClampingZeroOutDataTypeStr=Inherit: Inherit via back propagation  ClampingZeroOutMin=[]  ClampingZeroOutMax=[]  FilterDenConstantOutDataTypeStr=Inherit: Inherit via back propagation  FilterDenConstantOutMin=[]  FilterDenConstantOutMax=[]  PCopyOutDataTypeStr=Inherit: Inherit via back propagation  PCopyOutMin=[]  PCopyOutMax=[]  NCopyOutDataTypeStr=Inherit: Inherit via back propagation  NCopyOutMin=[]  NCopyOutMax=[]  IntegratorContinuousStateAttributes=''  IntegratorStateMustResolveToSignalObject=off  IntegratorRTWStateStorageClass=Auto  FilterContinuousStateAttributes=''  FilterStateMustResolveToSignalObject=off  FilterRTWStateStorageClass=Auto  ParallelPVariant=InternalParameters  IdealPVariant=Disabled  IVariant=InternalParameters  DVariant=Disabled  IntegratorVariant=Discrete  SatVariant=Disabled  AWVariant=Passthrough  PCopyVariant=Disabled  TRVariant=Disabled  FdbkBlocksVariant=Forward  IdealPFdbkVariant=Disabled  SatFdbkVariant=Disabled  DerivativeFilterVariant=Disabled  NVariant=Disabled  NCopyVariant=Disabled_SignalSpec  FilterICVariant=Disabled  IntegratorICVariant=InternalICs  ExternalResetVariant=Disabled  TRSumVariant=Passthrough  SumFdbkVariant=Disabled  SumVariant=Sum_PI  TsampFilterVariant=InternalTs  TsampNgainVariant=Passthrough  TsampIntegralVariant=Passthrough  ExternalSaturationOutDataTypeStr=Inherit: Same as second input
  PID Controller2 : slpidlib/PID Controller  Controller=PI  Form=Parallel  TimeDomain=Discrete-time  UseExternalTs=off  SampleTime=-1  IntegratorMethod=Forward Euler  FilterMethod=Forward Euler  ControllerParametersSource=internal  P=10  I=50  UseKiTs=off  D=0  N=100  UseFilter=on  TunerSelectOption=Transfer Function Based (PID Tuner App)  InitialConditionSource=internal  InitialConditionForIntegrator=0  InitialConditionForFilter=0  DifferentiatorICPrevScaledInput=0  ExternalReset=none  TrackingMode=off  Kt=1  LimitOutput=off  SatLimitsSource=internal  UpperSaturationLimit=inf  LowerSaturationLimit=-inf  LinearizeAsGain=on  AntiWindupMode=none  Kb=1  LimitIntegrator=off  UpperIntegratorSaturationLimit=inf  LowerIntegratorSaturationLimit=-inf  POutMin=[]  POutMax=[]  IOutMin=[]  IOutMax=[]  DOutMin=[]  DOutMax=[]  NOutMin=[]  NOutMax=[]  SumOutMin=[]  SumOutMax=[]  SaturationOutMin=[]  SaturationOutMax=[]  PParamMin=[]  PParamMax=[]  IParamMin=[]  IParamMax=[]  DParamMin=[]  DParamMax=[]  NParamMin=[]  NParamMax=[]  KbParamMin=[]  KbParamMax=[]  KtParamMin=[]  KtParamMax=[]  KbOutMin=[]  KbOutMax=[]  KtOutMin=[]  KtOutMax=[]  IntegratorOutMin=[]  IntegratorOutMax=[]  FilterOutMin=[]  FilterOutMax=[]  SumI1OutMin=[]  SumI1OutMax=[]  SumI2OutMin=[]  SumI2OutMax=[]  SumI3OutMin=[]  SumI3OutMax=[]  SumI4OutMin=[]  SumI4OutMax=[]  SumDOutMin=[]  SumDOutMax=[]  DifferentiatorOutMin=[]  DifferentiatorOutMax=[]  FilterDiffOutCoefMin=[]  FilterDiffOutCoefMax=[]  ReciprocalOutMin=[]  ReciprocalOutMax=[]  SumDenOutMin=[]  SumDenOutMax=[]  SumNumOutMin=[]  SumNumOutMax=[]  DivideOutMin=[]  DivideOutMax=[]  UdiffTsProdOutMin=[]  UdiffTsProdOutMax=[]  NTsProdOutMin=[]  NTsProdOutMax=[]  UintegralTsProdOutMin=[]  UintegralTsProdOutMax=[]  UngainTsProdOutMin=[]  UngainTsProdOutMax=[]  ClampingZeroOutDataTypeStr=Inherit: Inherit via back propagation  ClampingZeroOutMin=[]  ClampingZeroOutMax=[]  FilterDenConstantOutDataTypeStr=Inherit: Inherit via back propagation  FilterDenConstantOutMin=[]  FilterDenConstantOutMax=[]  PCopyOutDataTypeStr=Inherit: Inherit via back propagation  PCopyOutMin=[]  PCopyOutMax=[]  NCopyOutDataTypeStr=Inherit: Inherit via back propagation  NCopyOutMin=[]  NCopyOutMax=[]  IntegratorContinuousStateAttributes=''  IntegratorStateMustResolveToSignalObject=off  IntegratorRTWStateStorageClass=Auto  FilterContinuousStateAttributes=''  FilterStateMustResolveToSignalObject=off  FilterRTWStateStorageClass=Auto  ParallelPVariant=InternalParameters  IdealPVariant=Disabled  IVariant=InternalParameters  DVariant=Disabled  IntegratorVariant=Discrete  SatVariant=Disabled  AWVariant=Passthrough  PCopyVariant=Disabled  TRVariant=Disabled  FdbkBlocksVariant=Forward  IdealPFdbkVariant=Disabled  SatFdbkVariant=Disabled  DerivativeFilterVariant=Disabled  NVariant=Disabled  NCopyVariant=Disabled_SignalSpec  FilterICVariant=Disabled  IntegratorICVariant=InternalICs  ExternalResetVariant=Disabled  TRSumVariant=Passthrough  SumFdbkVariant=Disabled  SumVariant=Sum_PI  TsampFilterVariant=InternalTs  TsampNgainVariant=Passthrough  TsampIntegralVariant=Passthrough  ExternalSaturationOutDataTypeStr=Inherit: Same as second input
  PID Controller3 : slpidlib/PID Controller  Controller=PI  Form=Parallel  TimeDomain=Discrete-time  UseExternalTs=off  SampleTime=-1  IntegratorMethod=Forward Euler  FilterMethod=Forward Euler  ControllerParametersSource=internal  P=20  I=50  UseKiTs=off  D=0  N=100  UseFilter=on  TunerSelectOption=Transfer Function Based (PID Tuner App)  InitialConditionSource=internal  InitialConditionForIntegrator=0  InitialConditionForFilter=0  DifferentiatorICPrevScaledInput=0  ExternalReset=none  TrackingMode=off  Kt=1  LimitOutput=off  SatLimitsSource=internal  UpperSaturationLimit=inf  LowerSaturationLimit=-inf  LinearizeAsGain=on  AntiWindupMode=none  Kb=1  LimitIntegrator=off  UpperIntegratorSaturationLimit=inf  LowerIntegratorSaturationLimit=-inf  POutMin=[]  POutMax=[]  IOutMin=[]  IOutMax=[]  DOutMin=[]  DOutMax=[]  NOutMin=[]  NOutMax=[]  SumOutMin=[]  SumOutMax=[]  SaturationOutMin=[]  SaturationOutMax=[]  PParamMin=[]  PParamMax=[]  IParamMin=[]  IParamMax=[]  DParamMin=[]  DParamMax=[]  NParamMin=[]  NParamMax=[]  KbParamMin=[]  KbParamMax=[]  KtParamMin=[]  KtParamMax=[]  KbOutMin=[]  KbOutMax=[]  KtOutMin=[]  KtOutMax=[]  IntegratorOutMin=[]  IntegratorOutMax=[]  FilterOutMin=[]  FilterOutMax=[]  SumI1OutMin=[]  SumI1OutMax=[]  SumI2OutMin=[]  SumI2OutMax=[]  SumI3OutMin=[]  SumI3OutMax=[]  SumI4OutMin=[]  SumI4OutMax=[]  SumDOutMin=[]  SumDOutMax=[]  DifferentiatorOutMin=[]  DifferentiatorOutMax=[]  FilterDiffOutCoefMin=[]  FilterDiffOutCoefMax=[]  ReciprocalOutMin=[]  ReciprocalOutMax=[]  SumDenOutMin=[]  SumDenOutMax=[]  SumNumOutMin=[]  SumNumOutMax=[]  DivideOutMin=[]  DivideOutMax=[]  UdiffTsProdOutMin=[]  UdiffTsProdOutMax=[]  NTsProdOutMin=[]  NTsProdOutMax=[]  UintegralTsProdOutMin=[]  UintegralTsProdOutMax=[]  UngainTsProdOutMin=[]  UngainTsProdOutMax=[]  ClampingZeroOutDataTypeStr=Inherit: Inherit via back propagation  ClampingZeroOutMin=[]  ClampingZeroOutMax=[]  FilterDenConstantOutDataTypeStr=Inherit: Inherit via back propagation  FilterDenConstantOutMin=[]  FilterDenConstantOutMax=[]  PCopyOutDataTypeStr=Inherit: Inherit via back propagation  PCopyOutMin=[]  PCopyOutMax=[]  NCopyOutDataTypeStr=Inherit: Inherit via back propagation  NCopyOutMin=[]  NCopyOutMax=[]  IntegratorContinuousStateAttributes=''  IntegratorStateMustResolveToSignalObject=off  IntegratorRTWStateStorageClass=Auto  FilterContinuousStateAttributes=''  FilterStateMustResolveToSignalObject=off  FilterRTWStateStorageClass=Auto  ParallelPVariant=InternalParameters  IdealPVariant=Disabled  IVariant=InternalParameters  DVariant=Disabled  IntegratorVariant=Discrete  SatVariant=Disabled  AWVariant=Passthrough  PCopyVariant=Disabled  TRVariant=Disabled  FdbkBlocksVariant=Forward  IdealPFdbkVariant=Disabled  SatFdbkVariant=Disabled  DerivativeFilterVariant=Disabled  NVariant=Disabled  NCopyVariant=Disabled_SignalSpec  FilterICVariant=Disabled  IntegratorICVariant=InternalICs  ExternalResetVariant=Disabled  TRSumVariant=Passthrough  SumFdbkVariant=Disabled  SumVariant=Sum_PI  TsampFilterVariant=InternalTs  TsampNgainVariant=Passthrough  TsampIntegralVariant=Passthrough  ExternalSaturationOutDataTypeStr=Inherit: Same as second input
  PLL (3ph) : spsPLL3phLib/PLL (3ph)  Fmin=45  Par_Init=[0, 50]  ParK=[180, 3200, 1]  TcD=1e-4  MaxRateChangeFreq=12  FilterCutOffFreq=25  Ts=1/fsw  AGC=on
  PWM Generator (2-Level) : spsPWMGenerator2LevelLib/PWM Generator (2-Level)  ModulatorType=Three-phase bridge (6 pulses)  ModulatorMode=Unsynchronized  Fc=fsw  Pc=90  nF=27  MinMax="[ -1  1 ]"  SamplingTechnique=Natural  ModulatingSignals=off  m=0.8  Freq=60  Phase=0  Ts=Ts  ShowCarrierOutport=off
  Power (Positive-Sequence) : spsPowerPositiveSequenceLib/Power (Positive-Sequence)  Freq=50  Vinit=[0, 0]  Iinit=[0, 0]  Ts=1/fsw
      settings: LibrarySourceBlock=|
      | sps_lib/Sensors and Measurements/Power
      | (Positive-Sequence)
  Scope{,1..3} (4 alike) : Scope  NumInputPorts=2
  Scope{4,6..8} (4 alike) : Scope
  Scope5 : Scope  NumInputPorts=3
  Sum{,1..2,4,6} (5 alike) : Sum  Inputs=|+-
  Sum3 : Sum  Inputs=+|+|-
  Sum5 : Sum  Inputs=+|+
  Sum7 : Sum  Inputs=+|+|+
  dq0 to abc : spsdq0toabcLib/dq0 to abc  Alignment=90 degrees behind phase A axis
  gate : Outport
  wires:
  Constant/1 -> Mux/3
  PID Controller2/1 -> Sum5/2
  wt/1 -> dq0 to abc/2
  Mux/1 -> dq0 to abc/1
  Ud_ref/1 -> Scope/1, Sum/1
  Iq/1 -> Gain1/1, Sum6/2, Scope3/2
  Uq/1 -> Sum4/2, Scope1/2, Sum7/3, Gain3/1
  Sum3/1 -> Mux/1
  Sum5/1 -> Scope3/1, Sum6/1  "iq_ref"
  Sum2/1 -> PID Controller1/1
  Sum/1 -> PID Controller/1
  Sum7/1 -> Mux/2
  PID Controller1/1 -> Sum3/2  "Idef"
  Gain/1 -> Sum5/1
  Uq_ref/1 -> Scope1/1, Sum4/1
  Ud/1 -> Scope/2, Sum/2, Sum3/1, Gain/1
  Sum6/1 -> PID Controller3/1
  Sum4/1 -> PID Controller2/1
  Id/1 -> Gain4/1, Sum2/2, Scope2/2
  PID Controller3/1 -> Sum7/2  "Idef"
  PWM Generator (2-Level)/1 -> gate/1
  dq0 to abc/1 -> Gain2/1
  Gain2/1 -> Scope4/1, PWM Generator (2-Level)/1
  PID Controller/1 -> Sum1/1
  Gain3/1 -> Sum1/2
  Sum1/1 -> Scope2/1, Sum2/1
  Gain1/1 -> Sum3/3
  Gain4/1 -> Sum7/1
  PLL (3ph)/1 -> Scope8/1
  [Iabc] -> Power (Positive-Sequence)/2
  Demux3/1 -> Scope5/1
  Demux3/2 -> Scope5/2
  Power (Positive-Sequence)/1 -> Display1/1, Scope6/1
  [Uabc] -> PLL (3ph)/1, Power (Positive-Sequence)/1, Demux3/1
  Power (Positive-Sequence)/2 -> Display2/1, Scope7/1
  Demux3/3 -> Scope5/3

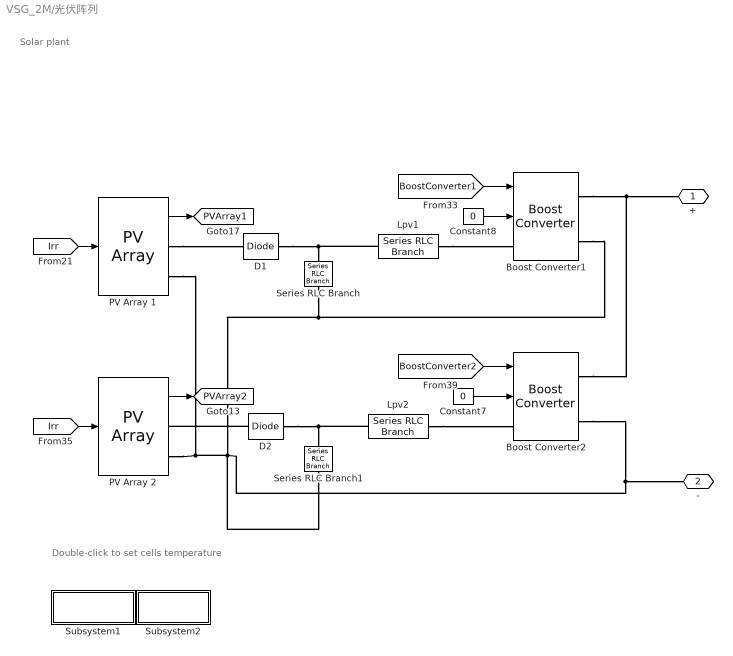
== system VSG_2M/光伏阵列 ==
  note: Solar plant
  note: Double-click to set cells temperature
  Boost Converter1 : spsBoostConverterLib/Boost Converter  ModelType=Switching devices  Ron=1e-4  Rs=1e6  Cs=inf  Vforward=[0,0]  Ron_Diode=1e-4  Rs_Diode=1e6  Cs_Diode=inf  Vf_Diode=0  Rs_CurrentSource=inf  Ron_ACsource=1e-3
      settings: LibrarySourceBlock=sps_lib/Power Electronics/Boost Converter
  Boost Converter2 : spsBoostConverterLib/Boost Converter  ModelType=Switching devices  Ron=1e-4  Rs=1e6  Cs=inf  Vforward=[0,0]  Ron_Diode=1e-4  Rs_Diode=1e6  Cs_Diode=inf  Vf_Diode=0  Rs_CurrentSource=inf  Ron_ACsource=1e-3
      settings: LibrarySourceBlock=sps_lib/Power Electronics/Boost Converter
  Constant7 : Constant  Value=0  SampleTime=Ts
  Constant8 : Constant  Value=0  SampleTime=Ts
  D1 : spsDiodeLib/Diode  Ron=1e-4  Lon=0  Vf=0  IC=0  UseSnubber=0  Rs=1e6  Cs=inf  Measurements=off
  D2 : spsDiodeLib/Diode  Ron=1e-4  Lon=0  Vf=0  IC=0  UseSnubber=0  Rs=1e6  Cs=inf  Measurements=off
  Lpv1 : spsSeriesRLCBranchLib/Series RLC Branch  LConnTagsString=__new0  RConnTagsString=__new0  BranchType=RL  Resistance=1e-3  Inductance=1e-3  SetiL0=off  InitialCurrent=0  Capacitance=120e-3  Setx0=off  InitialVoltage=0  Measurements=None
  Lpv2 : spsSeriesRLCBranchLib/Series RLC Branch  LConnTagsString=__new0  RConnTagsString=__new0  BranchType=RL  Resistance=1e-3  Inductance=1e-3  SetiL0=off  InitialCurrent=0  Capacitance=120e-3  Setx0=off  InitialVoltage=0  Measurements=None
  PV Array 1 : spsPVArrayLib/PV Array  Npar=282  Nser=15  PlotType=array @ 1000 W/m2 & specified temperatures  S_vec=[ 1000 250]  Temp_C_vec="[ 45 25  ]"  ModuleName=User-defined  PlotWhenSelected=off  Pm=355.012  Ncell=83  Voc=51.9  Isc=8.68  Vm=43.4  Im=8.18  beta_Voc_pc=-0.304  alpha_Isc_pc=0.017  beta_Voc=-0.15778  alpha_Isc=0.0014756  IL=8.6865  I0=3.3093e-11  nI=0.92618  Rsh=389.4331  Rs=0.29289  RobustModel=on  RobustCellTemperature=25  BAL=on  Tc=1e-6  Tfilter=5e-5
      settings: AttributesFormatString=(%<RobustCellTemperature> deg. C)
  PV Array 2 : spsPVArrayLib/PV Array  Npar=122  Nser=14  PlotType=array @ 1000 W/m2 & specified temperatures  S_vec=[ 1000 250]  Temp_C_vec="[ 45 25  ]"  ModuleName=User-defined  PlotWhenSelected=off  Pm=293.664  Ncell=60  Voc=39.5  Isc=9.60  Vm=32.2  Im=9.12  beta_Voc_pc=-0.300  alpha_Isc_pc=0.03  beta_Voc=-0.1185  alpha_Isc=0.00288  IL=9.6627  I0=3.1923e-11  nI=0.96973  Rsh=336.4947  Rs=0.3029  RobustModel=on  RobustCellTemperature=25  BAL=on  Tc=1e-6  Tfilter=5e-5
      settings: AttributesFormatString=(%<RobustCellTemperature> deg. C)
  Series RLC Branch : spsSeriesRLCBranchLib/Series RLC Branch  LConnTagsString=__new0  RConnTagsString=__new0  BranchType=C  Resistance=1  Inductance=1e-3  SetiL0=off  InitialCurrent=0  Capacitance=200e-6  Setx0=on  InitialVoltage=650  Measurements=None
  Series RLC Branch1 : spsSeriesRLCBranchLib/Series RLC Branch  LConnTagsString=__new0  RConnTagsString=__new0  BranchType=C  Resistance=1  Inductance=1e-3  SetiL0=off  InitialCurrent=0  Capacitance=200e-6  Setx0=on  InitialVoltage=450  Measurements=None
  Subsystem1 : Subsystem
      settings: OpenFcn=|
      | SystemName1=gcs;
      | BlockName1=[SystemName1, '/', 'PV Array 1'];
      | set_param(BlockName1,'RobustCellTemperature','25');
      | set_param(BlockName1,'ForegroundColor','black');
      | BlockName2=[SystemName1, '/', 'PV Array 2'];
      | set_param(BlockName2,'RobustCellTemperature','25');
      | set_param(BlockName2,'ForegroundColor','black');
      mask Display: disp('25 deg. C')
  Subsystem2 : Subsystem
      settings: OpenFcn=|
      | SystemName1=gcs;
      | BlockName1=[SystemName1, '/', 'PV Array 1'];
      | set_param(BlockName1,'RobustCellTemperature','45');
      | set_param(BlockName1,'ForegroundColor','red');
      | BlockName2=[SystemName1, '/', 'PV Array 2'];
      | set_param(BlockName2,'RobustCellTemperature','45');
      | set_param(BlockName2,'ForegroundColor','red');
      mask Display: disp('45 deg. C')
  + : PMIOPort  Side=Right
  - : PMIOPort  Port=2  Side=Right
  tag scope: PVArray1=global, PVArray2=global
  wires:
  [BoostConverter2] -> Boost Converter2/1
  [BoostConverter1] -> Boost Converter1/1
  PV Array 1/1 -> [PVArray1]
  PV Array 2/1 -> [PVArray2]
  [Irr] -> PV Array 2/1
  Constant8/1 -> Boost Converter1/2
  [Irr] -> PV Array 1/1
  Constant7/1 -> Boost Converter2/2
  connections:
  D1/RConn1 -- Series RLC Branch/LConn1 -- Lpv1/RConn1
  Boost Converter1/RConn1 -- Boost Converter2/RConn1 -- +/RConn1
  Series RLC Branch1/RConn1 -- PV Array 2/RConn2 -- PV Array 1/RConn2 -- Series RLC Branch/RConn1 -- Boost Converter1/RConn2 -- Boost Converter2/RConn2 -- -/RConn1
  D2/RConn1 -- Series RLC Branch1/LConn1 -- Lpv2/RConn1
  Lpv2/LConn1 -- Boost Converter2/LConn1
  PV Array 1/RConn1 -- D1/LConn1
  Lpv1/LConn1 -- Boost Converter1/LConn1
  D2/LConn1 -- PV Array 2/RConn1

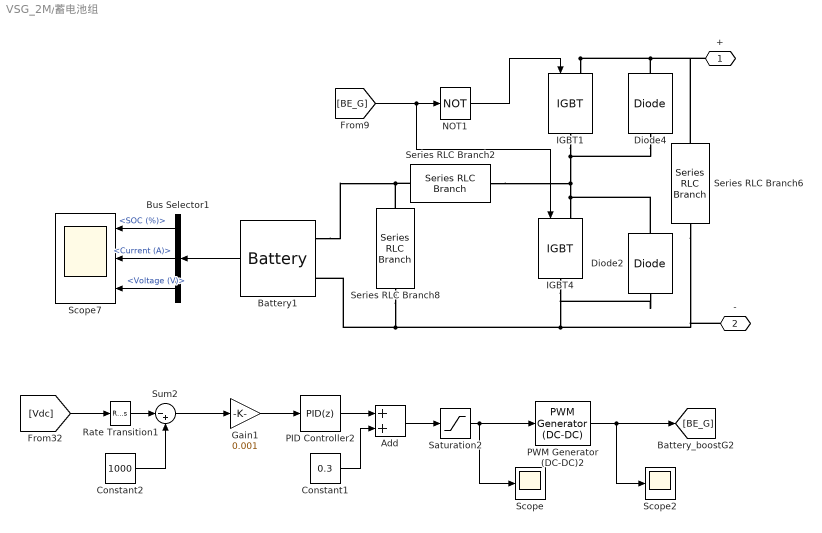
== system VSG_2M/蓄电池组 ==
  Add : Sum
  Battery1 : spsBatteryLib/Battery  BatType=Lithium-Ion  ShowTempParam=off  ThermalPreset=no  ShowAgeParam=off  NomV=300  NomQ=100  SOC=100  Batt_Tr=0.1  PresetModel=on  MaxQ=100  MinV=225  FullV=349.1961  Dis_rate=43.4783  R=0.03  Normal_OP=90.4348  expZone="[324.1158      4.913043]"  current=[6.5 13 32.5]  Units=Time  Tci=20  NomT=20  T2=-30  MaxQ2=4.8  FullV2=7.1  Normal_OP2=5.655  expZone2="[6.58           1]"  Rca=0.6  ti=2000  Dp=0  Neq0=0  Tsim=1e6  Ta1=25  Qeol=5.4*0.9  Reol=0.013333*1.2  Char_age=[2.3478, 3]  Dis_age=[2.3478, 10]  N1=1500  N2=10500  N3=1000  N4=1400  Ta2=45  N5=950
  Bus Selector1 : BusSelector  OutputSignals=SOC (%),Current (A),Voltage (V)
  Constant1 : Constant  Value=0.3
  Constant2 : Constant  Value=1000
  Diode2 : spsDiodeLib/Diode  Ron=0.001  Lon=0  Vf=0.8  IC=0  UseSnubber=off  Rs=500  Cs=250e-9  Measurements=off
  Diode4 : spsDiodeLib/Diode  Ron=0.001  Lon=0  Vf=0.8  IC=0  UseSnubber=off  Rs=500  Cs=250e-9  Measurements=off
  Gain1 : Gain  Gain=0.001
  IGBT1 : spsIGBTLib/IGBT  Ron=0.001  Lon=0  Vf=1  Tf=1e-6  Tt=2e-6  IC=0  Rs=1e5  Cs=inf  Measurements=off
  IGBT4 : spsIGBTLib/IGBT  Ron=0.001  Lon=0  Vf=1  Tf=1e-6  Tt=2e-6  IC=0  Rs=1e5  Cs=inf  Measurements=off
  NOT1 : Logic  Operator=NOT  IconShape=distinctive  AllPortsSameDT=off  OutDataTypeStr=boolean
  PID Controller2 : slpidlib/PID Controller  Controller=PID  Form=Parallel  TimeDomain=Discrete-time  UseExternalTs=off  SampleTime=-1  IntegratorMethod=Forward Euler  FilterMethod=Forward Euler  ControllerParametersSource=internal  P=2  I=4  UseKiTs=off  D=0.008  N=100  UseFilter=on  TunerSelectOption=Transfer Function Based (PID Tuner App)  InitialConditionSource=internal  InitialConditionForIntegrator=0  InitialConditionForFilter=0  DifferentiatorICPrevScaledInput=0  ExternalReset=none  TrackingMode=off  Kt=1  LimitOutput=off  SatLimitsSource=internal  UpperSaturationLimit=0.1  LowerSaturationLimit=-0.1  LinearizeAsGain=off  AntiWindupMode=clamping  Kb=1  LimitIntegrator=off  UpperIntegratorSaturationLimit=5  LowerIntegratorSaturationLimit=-5  POutMin=[]  POutMax=[]  IOutMin=[]  IOutMax=[]  DOutMin=[]  DOutMax=[]  NOutMin=[]  NOutMax=[]  SumOutMin=[]  SumOutMax=[]  SaturationOutMin=[]  SaturationOutMax=[]  PParamMin=[]  PParamMax=[]  IParamMin=[]  IParamMax=[]  DParamMin=[]  DParamMax=[]  NParamMin=[]  NParamMax=[]  KbParamMin=[]  KbParamMax=[]  KtParamMin=[]  KtParamMax=[]  KbOutMin=[]  KbOutMax=[]  KtOutMin=[]  KtOutMax=[]  IntegratorOutMin=[]  IntegratorOutMax=[]  FilterOutMin=[]  FilterOutMax=[]  SumI1OutMin=[]  SumI1OutMax=[]  SumI2OutMin=[]  SumI2OutMax=[]  SumI3OutMin=[]  SumI3OutMax=[]  SumI4OutMin=[]  SumI4OutMax=[]  SumDOutMin=[]  SumDOutMax=[]  DifferentiatorOutMin=[]  DifferentiatorOutMax=[]  FilterDiffOutCoefMin=[]  FilterDiffOutCoefMax=[]  ReciprocalOutMin=[]  ReciprocalOutMax=[]  SumDenOutMin=[]  SumDenOutMax=[]  SumNumOutMin=[]  SumNumOutMax=[]  DivideOutMin=[]  DivideOutMax=[]  UdiffTsProdOutMin=[]  UdiffTsProdOutMax=[]  NTsProdOutMin=[]  NTsProdOutMax=[]  UintegralTsProdOutMin=[]  UintegralTsProdOutMax=[]  UngainTsProdOutMin=[]  UngainTsProdOutMax=[]  ClampingZeroOutDataTypeStr=Inherit: Inherit via back propagation  ClampingZeroOutMin=[]  ClampingZeroOutMax=[]  FilterDenConstantOutDataTypeStr=Inherit: Inherit via back propagation  FilterDenConstantOutMin=[]  FilterDenConstantOutMax=[]  PCopyOutDataTypeStr=Inherit: Inherit via back propagation  PCopyOutMin=[]  PCopyOutMax=[]  NCopyOutDataTypeStr=Inherit: Inherit via back propagation  NCopyOutMin=[]  NCopyOutMax=[]  IntegratorContinuousStateAttributes=''  IntegratorStateMustResolveToSignalObject=off  IntegratorRTWStateStorageClass=Auto  FilterContinuousStateAttributes=''  FilterStateMustResolveToSignalObject=off  FilterRTWStateStorageClass=Auto  ParallelPVariant=InternalParameters  IdealPVariant=Disabled  IVariant=InternalParameters  DVariant=InternalParameters  IntegratorVariant=Discrete  SatVariant=Disabled  AWVariant=Passthrough  PCopyVariant=Disabled  TRVariant=Disabled  FdbkBlocksVariant=Forward  IdealPFdbkVariant=Disabled  SatFdbkVariant=Disabled  DerivativeFilterVariant=ForwardEulerFilter  NVariant=InternalParameters  NCopyVariant=Disabled  FilterICVariant=InternalICsFilter  IntegratorICVariant=InternalICs  ExternalResetVariant=Disabled  TRSumVariant=Passthrough  SumFdbkVariant=Disabled  SumVariant=Sum_PID  TsampFilterVariant=InternalTs  TsampNgainVariant=Passthrough  TsampIntegralVariant=Passthrough  ExternalSaturationOutDataTypeStr=Inherit: Same as second input
  PWM Generator (DC-DC)2 : spsPWMGeneratorDCDCLib/PWM Generator (DC-DC)  Fsw=10000  Ts=0
  Rate Transition1 : RateTransition  OutPortSampleTime=50e-6
  Saturation2 : Saturate  UpperLimit=0.9  LowerLimit=0.01
  Scope : Scope
  Scope2 : Scope
  Scope7 : Scope  NumInputPorts=3
  Series RLC Branch2 : spsSeriesRLCBranchLib/Series RLC Branch  LConnTagsString=__new0  RConnTagsString=__new0  BranchType=L  Resistance=1  Inductance=0.002  SetiL0=off  InitialCurrent=0  Capacitance=1e-6  Setx0=off  InitialVoltage=0  Measurements=None
  Series RLC Branch6 : spsSeriesRLCBranchLib/Series RLC Branch  LConnTagsString=__new0  RConnTagsString=__new0  BranchType=C  Resistance=1  Inductance=1e-3  SetiL0=off  InitialCurrent=0  Capacitance=470e-4  Setx0=off  InitialVoltage=0  Measurements=None
  Series RLC Branch8 : spsSeriesRLCBranchLib/Series RLC Branch  LConnTagsString=__new0  RConnTagsString=__new0  BranchType=C  Resistance=1  Inductance=1e-3  SetiL0=off  InitialCurrent=0  Capacitance=470e-6  Setx0=off  InitialVoltage=0  Measurements=None
  Sum2 : Sum  Inputs=|-+
  + : PMIOPort  Side=Right
  - : PMIOPort  Port=2  Side=Right
  wires:
  Saturation2/1 -> Scope/1, PWM Generator (DC-DC)2/1
  Bus Selector1/2 -> Scope7/2  "<Current (A)>"
  Rate Transition1/1 -> Sum2/1
  Constant2/1 -> Sum2/2
  Add/1 -> Saturation2/1
  Constant1/1 -> Add/2
  [BE_G] -> IGBT4/1, NOT1/1
  Sum2/1 -> Gain1/1
  PID Controller2/1 -> Add/1
  Bus Selector1/1 -> Scope7/1  "<SOC (%)>"
  [Vdc] -> Rate Transition1/1
  Gain1/1 -> PID Controller2/1
  NOT1/1 -> IGBT1/1
  Battery1/1 -> Bus Selector1/1
  PWM Generator (DC-DC)2/1 -> Scope2/1, [BE_G]
  Bus Selector1/3 -> Scope7/3  "<Voltage (V)>"
  connections:
  IGBT1/RConn1 -- Diode4/LConn1 -- Series RLC Branch2/RConn1 -- Diode2/RConn1 -- IGBT4/LConn1
  Series RLC Branch2/LConn1 -- Series RLC Branch8/LConn1 -- Battery1/LConn1
  Series RLC Branch8/RConn1 -- Battery1/LConn2 -- Diode2/LConn1 -- IGBT4/RConn1 -- -/RConn1 -- Series RLC Branch6/RConn1
  IGBT1/LConn1 -- Diode4/RConn1 -- +/RConn1 -- Series RLC Branch6/LConn1

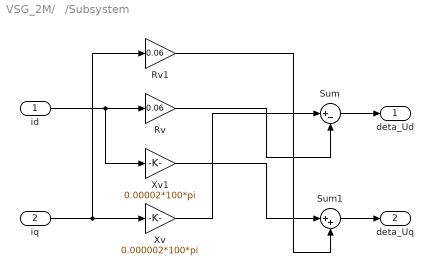
== system VSG_2M/   /Subsystem ==
  id : Inport
  iq : Inport  Port=2
  Rv : Gain  Gain=0.06
  Rv1 : Gain  Gain=0.06
  Sum : Sum  Inputs=|+-
  Sum1 : Sum  Inputs=|++
  Xv : Gain  Gain=0.000002*100*pi
  Xv1 : Gain  Gain=0.00002*100*pi
  deta_Ud : Outport
  deta_Uq : Outport  Port=2
  wires:
  Sum/1 -> deta_Ud/1
  Sum1/1 -> deta_Uq/1
  id/1 -> Xv1/1, Rv/1
  Rv/1 -> Sum/2
  iq/1 -> Rv1/1, Xv/1
  Xv/1 -> Sum/1
  Xv1/1 -> Sum1/1
  Rv1/1 -> Sum1/2
